simulink model "early_exit_same_level_2018a"  (R2018a)
settings: Solver=FixedStepDiscrete  StartTime=0.0  StopTime=10.0  FixedStep=0.1  RelTol=1e-3  EnableMultiTasking=on
settings Model: Creator=bzhan  LastModifiedBy=bzhan
settings SolverCC: AutoInsertRateTranBlk=on
settings DataIOCC: LimitDataPoints=on  ReturnWorkspaceOutputs=on
settings OptimizationCC: LifeSpan=inf
settings DebuggingCC: AllowSymbolicDim=off  SFUnexpectedBacktrackingDiag=warning  SFNoUnconditionalDefaultTransitionDiag=warning  SFExecutionAtInitializationDiag=none
settings CodeAppCC: StateflowObjectComments=on
settings GRTTargetCC: TargetLangStandard=C89/C90 (ANSI)
settings ConfigComp: CovMetricSettings=dw  CovHtmlReporting=on  CovSaveCumulativeToWorkspaceVar=on  CovSaveSingleToWorkspaceVar=on  CovShowResultsExplorer=off  CovExternalEMLEnable=off  CovSFcnEnable=off

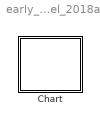
== system early_exit_same_level_2018a ==
  Chart : Stateflow chart  TreatAsAtomicUnit=on

== stateflow chart early_exit_same_level_2018a/Chart ==
  state A
    en: f("en_A")
    ex: f("ex_A")
  state B
    en: f("en_B")
    ex: f("ex_B")
  state C
    en: f("en_C")
    ex: f("ex_C")
  (default) -> A : {data = 1}
  A -> B [order 1] : [data==1]{data=2;E}
  A -> C [order 2] : E
  data: s function_input; data local
  events: E local FUNCTION_CALL_EVENT
  function f(s):
    | function f(s)
    |   fprintf(s+"\n");
